simulink model "Sim_exe"  (R2023b)
settings: Solver=VariableStepAuto  StartTime=0.0  StopTime=Tf  RelTol=1e-4  AbsTol=1e-4
values from neighbouring files (symbols this model uses):
  A = fx(x_f,u_f)    [Main.m]
  B = fu(x_f,u_f)    [Main.m]
  C = zeros(1,2)    [Main.m]
  D = zeros(2)    [Main.m]
  dCMax = 1    [Main.m]
  Ko = Ko'    [Main.m]
  u_f = w0^2*cos(th_f)*m*L^2    [Main.m]
  x_f = [thp_f; th_f]    [Main.m]
undefined symbols (not defined in the file or in its folder): K, Namp, Tamp, Tf, Tfreq, Wamp
settings Model: Creator=emanuele riva  LastModifiedBy=emanu
settings SolverCC: AutoScaleAbsTol=off  AlgebraicLoopSolver=TrustRegion
settings DataIOCC: ReturnWorkspaceOutputs=off
settings DebuggingCC: UnconnectedInputMsg=warning  UnconnectedOutputMsg=warning  UnconnectedLineMsg=warning  ArithmeticOperatorsInVariantConditions=warning
settings ModelReferenceCC: EnableRefExpFcnMdlSchedulingChecks=on
settings SFSimCC: SimUseLocalCustomCode=off  CustomCodeUndefinedFunction=UseInterfaceOnly
settings RTWCC: RTWUseLocalCustomCode=off  DLArmComputeVersion=19.05
settings CodeAppCC: StateflowObjectComments=on

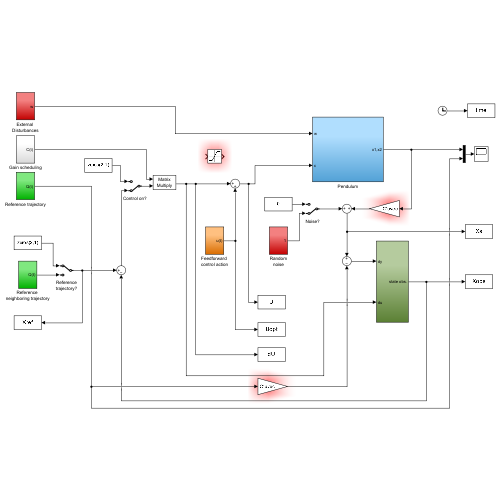
[thumbnail: Simulink's stored preview of the top-level diagram]
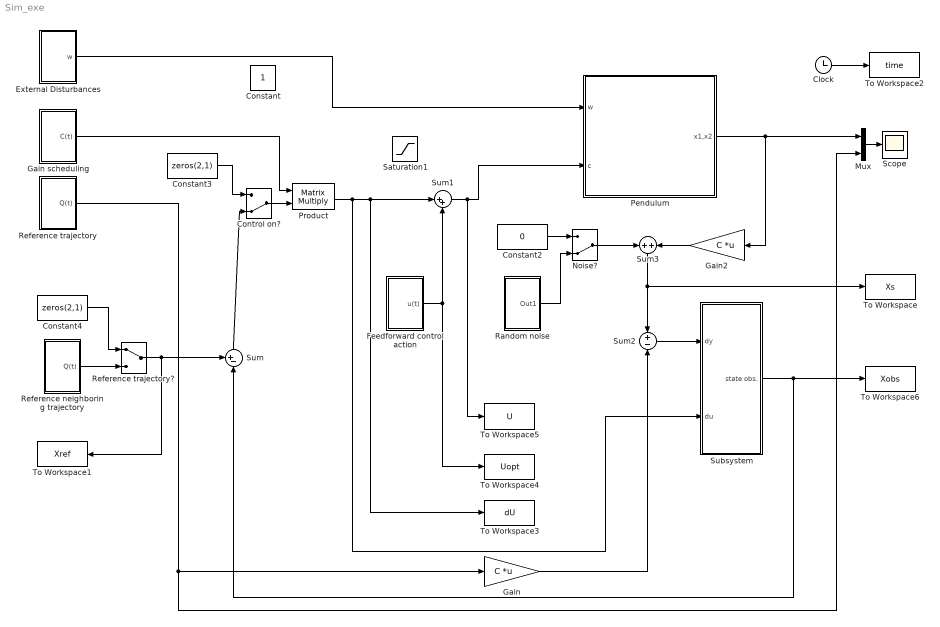
== system Sim_exe ==
  Clock : Clock
  Constant2 : Constant  Value=0  VectorParams1D=off
  Constant3 : Constant  Value=zeros(2,1)  VectorParams1D=off
  Constant4 : Constant  Value=zeros(2,1)  VectorParams1D=off
  Control on? : ManualSwitch  CurrentSetting=0
  External Disturbances : Subsystem
  Feedforward control action : Subsystem
  Gain : Gain  Gain=C  Multiplication=Matrix(K*u) (u vector)
  Gain scheduling : Subsystem
  Gain2 : Gain  Gain=C  Multiplication=Matrix(K*u) (u vector)
  Mux : Mux  Inputs=2
  Noise? : ManualSwitch  CurrentSetting=0
  Pendulum : Subsystem
  Product : Product  Multiplication=Matrix(*)
  Random noise : Subsystem
  Reference trajectory? : ManualSwitch
  Reference neighboring trajectory : Subsystem
  Reference trajectory : Subsystem
  Saturation1 : Saturate  UpperLimit=dCMax  LowerLimit=-dCMax
  Scope : Scope
  Subsystem : Subsystem
  Sum : Sum  Inputs=+-|
  Sum1 : Sum  Inputs=|++
  Sum2 : Sum  Inputs=+-
  Sum3 : Sum
  To Workspace : ToWorkspace  VariableName=Xs  SaveFormat=Timeseries  SampleTime=-1
  To Workspace1 : ToWorkspace  VariableName=Xref  SaveFormat=Timeseries  SampleTime=-1
  To Workspace2 : ToWorkspace  VariableName=time  SaveFormat=Timeseries  SampleTime=-1
  To Workspace3 : ToWorkspace  VariableName=dU  SaveFormat=Timeseries  SampleTime=-1
  To Workspace4 : ToWorkspace  VariableName=Uopt  SaveFormat=Timeseries  SampleTime=-1
  To Workspace5 : ToWorkspace  VariableName=U  SaveFormat=Timeseries  SampleTime=-1
  To Workspace6 : ToWorkspace  VariableName=Xobs  SaveFormat=Timeseries  SampleTime=-1
  Constant : Constant  IOType=siggen
  wires:
  Pendulum/1(x1,x2) -> Gain2/1, Mux/1
  Reference trajectory/1(Q(t)) -> Mux/2, Gain/1
  Gain scheduling/1(C(t)) -> Product/1
  Mux/1 -> Scope/1
  Clock/1 -> To Workspace2/1
  Feedforward control action/1(u(t)) -> Sum1/2, To Workspace4/1
  Sum1/1 -> Pendulum/2(c), To Workspace5/1
  Sum2/1 -> Subsystem/1(dy)
  Gain/1 -> Sum2/2
  Product/1 -> Sum1/1, To Workspace3/1, Subsystem/2(du)
  Subsystem/1(state obs.) -> To Workspace6/1, Sum/2
  Constant2/1 -> Noise?/1
  Random noise/1(Out1) -> Noise?/2
  Gain2/1 -> Sum3/2
  Noise?/1 -> Sum3/1
  Sum3/1 -> To Workspace/1, Sum2/1
  Constant3/1 -> Control on?/1
  Control on?/1 -> Product/2
  Constant4/1 -> Reference trajectory?/1
  Reference neighboring trajectory/1(Q(t)) -> Reference trajectory?/2
  Reference trajectory?/1 -> Sum/1, To Workspace1/1
  Sum/1 -> Control on?/2
  External Disturbances/1(w) -> Pendulum/1(w)

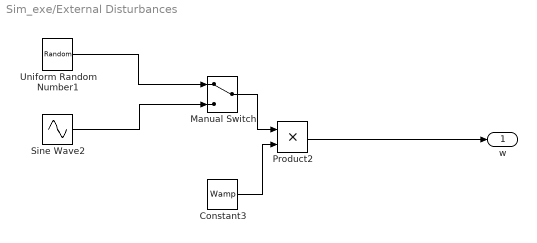
== system Sim_exe/External Disturbances ==
  Constant3 : Constant  Value=Wamp  VectorParams1D=off
  Manual Switch : ManualSwitch
  Product2 : Product
  Sine Wave2 : Sin  Frequency=2*pi*100  SampleTime=0  VectorParams1D=off
  Uniform Random Number1 : UniformRandomNumber  SampleTime=Tf/1000  VectorParams1D=off
  w : Outport
  wires:
  Sine Wave2/1 -> Manual Switch/2
  Manual Switch/1 -> Product2/1
  Uniform Random Number1/1 -> Manual Switch/1
  Constant3/1 -> Product2/2
  Product2/1 -> w/1

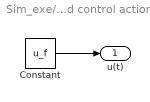
== system Sim_exe/Feedforward control action ==
  Constant : Constant  Value=u_f
  u(t) : Outport
  wires:
  Constant/1 -> u(t)/1

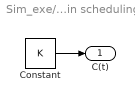
== system Sim_exe/Gain scheduling ==
  Constant : Constant  Value=K  VectorParams1D=off
  C(t) : Outport
  wires:
  Constant/1 -> C(t)/1

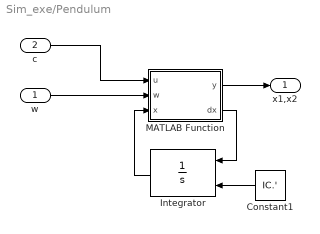
== system Sim_exe/Pendulum ==
  w : Inport
  c : Inport  Port=2
  Constant1 : Constant  Value=IC.'  VectorParams1D=off
  Integrator : Integrator  InitialConditionSource=external
  MATLAB Function : MATLAB Function  TreatAsAtomicUnit=on
  x1,x2 : Outport
  wires:
  MATLAB Function/2(dx) -> Integrator/1
  Integrator/1 -> MATLAB Function/3(x)
  Constant1/1 -> Integrator/2
  MATLAB Function/1(y) -> x1,x2/1
  c/1 -> MATLAB Function/1(u)
  w/1 -> MATLAB Function/2(w)

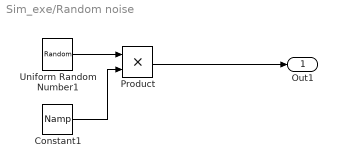
== system Sim_exe/Random noise ==
  Constant1 : Constant  Value=Namp  VectorParams1D=off
  Product : Product
  Uniform Random Number1 : UniformRandomNumber  Seed=19  SampleTime=0.001  VectorParams1D=off
  Out1 : Outport
  wires:
  Constant1/1 -> Product/2
  Uniform Random Number1/1 -> Product/1
  Product/1 -> Out1/1

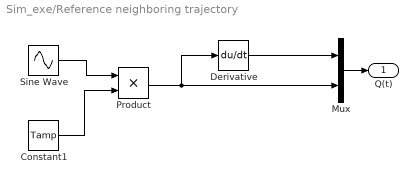
== system Sim_exe/Reference neighboring trajectory ==
  Constant1 : Constant  Value=Tamp  VectorParams1D=off
  Derivative : Derivative
  Mux : Mux  Inputs=2
  Product : Product
  Sine Wave : Sin  Frequency=Tfreq  SampleTime=0  VectorParams1D=off
  Q(t) : Outport
  wires:
  Sine Wave/1 -> Product/1
  Constant1/1 -> Product/2
  Mux/1 -> Q(t)/1
  Product/1 -> Mux/2, Derivative/1
  Derivative/1 -> Mux/1

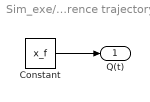
== system Sim_exe/Reference trajectory ==
  Constant : Constant  Value=x_f  VectorParams1D=off
  Q(t) : Outport
  wires:
  Constant/1 -> Q(t)/1

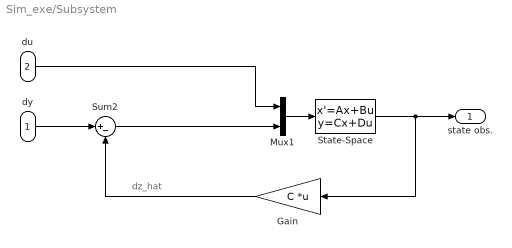
== system Sim_exe/Subsystem ==
  note: dz_hat
  dy : Inport
  du : Inport  Port=2
  Gain : Gain  Gain=C  Multiplication=Matrix(K*u) (u vector)
  Mux1 : Mux  Inputs=2
  State-Space : StateSpace  A=A  B=[B Ko]  C=eye(2,2)  D=D  InitialCondition=ICobs.'
  Sum2 : Sum  Inputs=|+-
  state obs. : Outport
  wires:
  Mux1/1 -> State-Space/1
  State-Space/1 -> state obs./1, Gain/1
  Gain/1 -> Sum2/2
  du/1 -> Mux1/1
  dy/1 -> Sum2/1
  Sum2/1 -> Mux1/2

== matlab function Sim_exe/Pendulum/MATLAB Function ==
  data: y output; dx output; u input; w input; x input
function [y,dx]  = fcn(u,w,x)

m = 1;
g = 9.81;
L = 0.1;
zeta = 0.02;
w0 = sqrt(g/L);

dx = zeros(2,1);

u = u(1) + w(1);

dx(1) = - 2*zeta*w0*x(1) - w0^2*sin(x(2)) + u/L^2/m;
dx(2) = x(1);

y = [x(1);x(2)];
